simulink model "LKA_RL_staliro"  (R2021a)
settings: Solver=FixedStepAuto  StartTime=0.0  StopTime=T  FixedStep=Ts  RelTol=1e-3
undefined symbols (not defined in the file): Cf, Cr, DiscIntNeverNeededParam, e1_initial, e2_initial, Iz, lf, lr, m, max_late_dev, md, terminate_error, Ts, u_max, u_min, Vx
libraries: rllib x1, simulink x1
settings Model: Creator=The MathWorks, Inc.  LastModifiedBy=ldy
settings SolverCC: AlgebraicLoopSolver=TrustRegion
settings DataIOCC: ReturnWorkspaceOutputs=off
settings DebuggingCC: SFMachineParentedDataDiag=warning  ArithmeticOperatorsInVariantConditions=warning
settings SFSimCC: SimUseLocalCustomCode=off  CustomCodeUndefinedFunction=UseInterfaceOnly
settings RTWCC: RTWUseLocalCustomCode=off
settings CodeAppCC: StateflowObjectComments=on
settings SimscapeCC: SimscapeNormalizeSystem=off

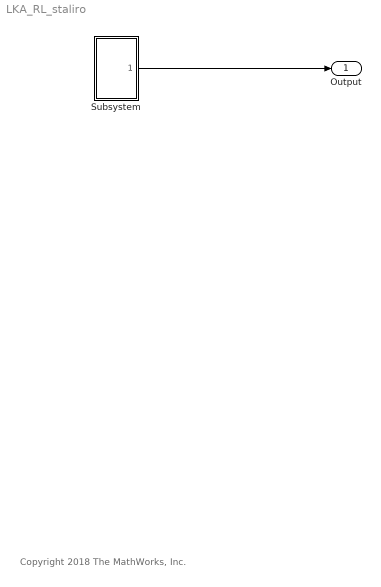
== system LKA_RL_staliro ==
  note: Copyright 2018 The MathWorks, Inc.
  Subsystem : Subsystem
  Output : Outport
  wires:
  Subsystem/1(Outport) -> Output/1

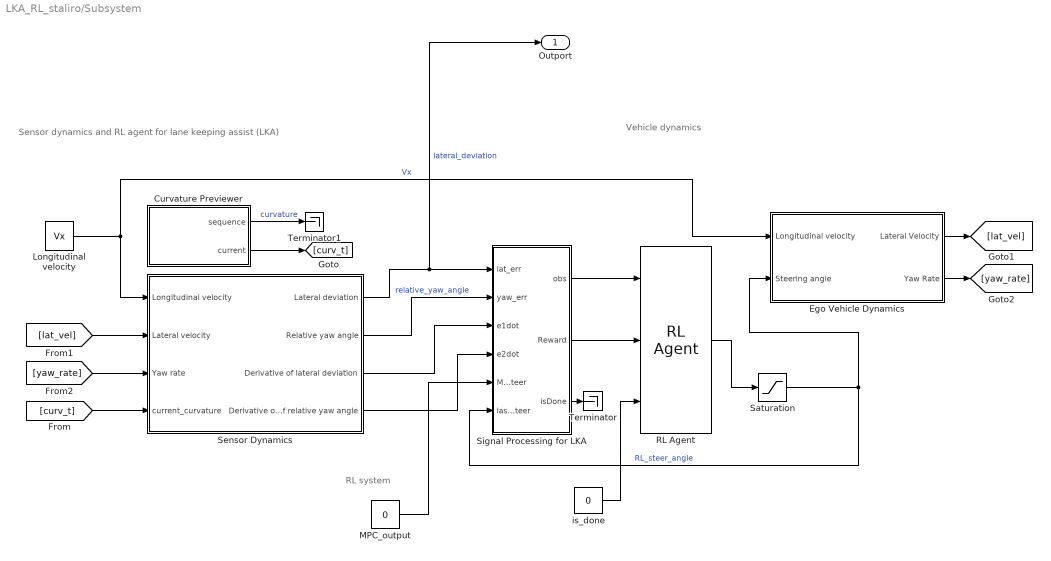
== system LKA_RL_staliro/Subsystem ==
  note: RL system
  note: Vehicle dynamics
  note: Sensor dynamics and RL agent for lane keeping assist (LKA)
  Curvature Previewer : Subsystem  mask{signal=md, ts=Ts, steps=10}
      mask prompts: signal "Signal name"; ts "Sampling time"; steps "Number of previewing steps"
      mask init:
      | ts = evalin('base',get_param(gcbh,'ts'));
      | signal = evalin('base',get_param(gcbh,'signal'));
      | steps = evalin('base',get_param(gcbh,'steps'));
      | data = mpc_previewer_maskinit(signal,ts);
      mask Display:
      | fprintf('Future\nsample\nextractor');
      | port_label('output', 1, 'seq')
      | port_label('output', 2, '@t')
  Ego Vehicle Dynamics : Subsystem
  Longitudinal velocity : Constant  Value=Vx  SampleTime=Ts
  MPC_output : Constant  Value=0
  RL Agent : rllib/RL Agent  Agent=agent  ExternalActionAsInput=off  ProvideCumRwd=off  TreatAsDirectFeedthrough=on
  Saturation : Saturate  UpperLimit=u_max  LowerLimit=u_min
  Sensor Dynamics : Subsystem
  "Signal Processing for LKA " : Subsystem
  Terminator : Terminator
  Terminator1 : Terminator
  is_done : Constant  Value=0
  Outport : Outport
  wires:
  Curvature Previewer/2(current) -> [curv_t]
  [curv_t] -> Sensor Dynamics/4(current_curvature)
  Curvature Previewer/1(sequence) -> Terminator1/1  "curvature"
  [yaw_rate] -> Sensor Dynamics/3(Yaw rate)
  Ego Vehicle Dynamics/1(Lateral Velocity) -> [lat_vel]
  MPC_output/1 -> "Signal Processing for LKA "/5(MPC_steer)
  is_done/1 -> RL Agent/3
  Sensor Dynamics/3(Derivative of lateral deviation) -> "Signal Processing for LKA "/3("e1dot ")
  "Signal Processing for LKA "/2(Reward) -> RL Agent/2
  Sensor Dynamics/1(Lateral deviation) -> Outport/1, "Signal Processing for LKA "/1(lat_err)  "lateral_deviation"
  RL Agent/1 -> Saturation/1
  "Signal Processing for LKA "/1(obs) -> RL Agent/1
  Sensor Dynamics/4(Derivative of relative yaw angle) -> "Signal Processing for LKA "/4(e2dot)
  [lat_vel] -> Sensor Dynamics/2(Lateral velocity)
  Saturation/1 -> "Signal Processing for LKA "/6(last_RL_steer), Ego Vehicle Dynamics/2(Steering angle)  "RL_steer_angle"
  Sensor Dynamics/2(Relative yaw angle) -> "Signal Processing for LKA "/2(yaw_err)  "relative_yaw_angle"
  Ego Vehicle Dynamics/2(Yaw Rate) -> [yaw_rate]
  Longitudinal velocity/1 -> Ego Vehicle Dynamics/1(Longitudinal velocity), Sensor Dynamics/1(Longitudinal velocity)  "Vx"
  "Signal Processing for LKA "/3(isDone) -> Terminator/1

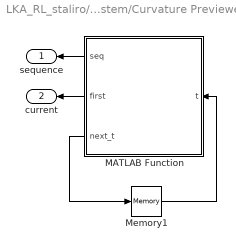
== system LKA_RL_staliro/Subsystem/Curvature Previewer ==
  MATLAB Function : MATLAB Function  TreatAsAtomicUnit=on
  Memory1 : Memory  InheritSampleTime=on  LinearizeAsDelay=on
  sequence : Outport  VectorParamsAs1DForOutWhenUnconnected=off
  current : Outport  Port=2  VectorParamsAs1DForOutWhenUnconnected=off
  wires:
  MATLAB Function/1(seq) -> sequence/1
  MATLAB Function/2(first) -> current/1
  Memory1/1 -> MATLAB Function/1(t)
  MATLAB Function/3(next_t) -> Memory1/1

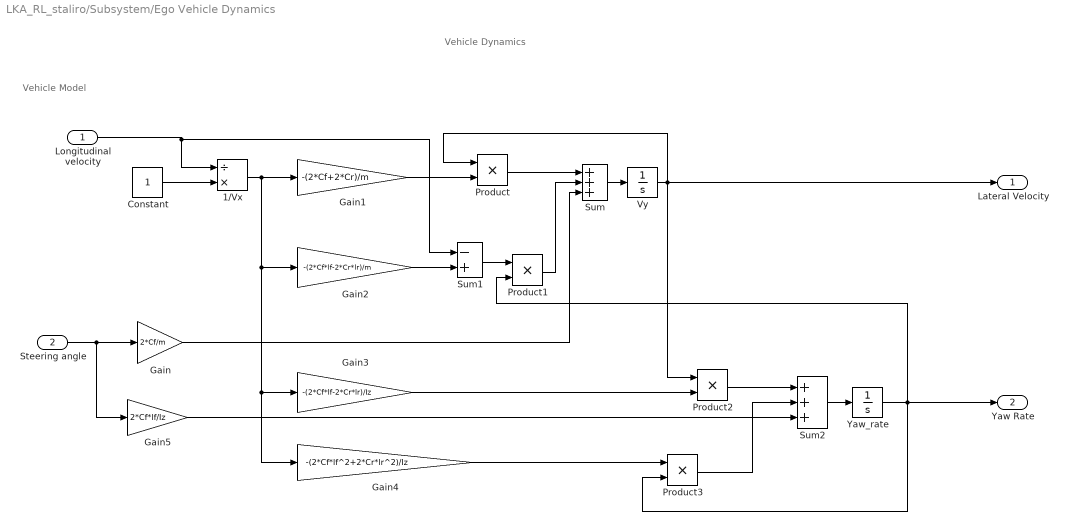
== system LKA_RL_staliro/Subsystem/Ego Vehicle Dynamics ==
  note: Vehicle Model
  note: Vehicle Dynamics
  Longitudinal velocity : Inport
  Steering angle : Inport  Port=2
  1/Vx : Product  Inputs=/*
  Constant : Constant
  Gain : Gain  Gain=2*Cf/m
  Gain1 : Gain  Gain=-(2*Cf+2*Cr)/m
  Gain2 : Gain  Gain=-(2*Cf*lf-2*Cr*lr)/m
  Gain3 : Gain  Gain=-(2*Cf*lf-2*Cr*lr)/Iz
  Gain4 : Gain  Gain=-(2*Cf*lf^2+2*Cr*lr^2)/Iz
  Gain5 : Gain  Gain=2*Cf*lf/Iz
  Product{,1..3} (4 alike) : Product
  Sum : Sum  Inputs=+++
  Sum1 : Sum  Inputs=-+
  Sum2 : Sum  Inputs=+++
  Vy : Integrator
  "Yaw_rate " : Integrator
  Lateral Velocity : Outport  VectorParamsAs1DForOutWhenUnconnected=off
  Yaw Rate : Outport  Port=2  VectorParamsAs1DForOutWhenUnconnected=off
  wires:
  Sum2/1 -> "Yaw_rate "/1
  Gain2/1 -> Sum1/2
  Gain4/1 -> Product3/1
  Constant/1 -> 1/Vx/2
  Gain3/1 -> Product2/2
  1/Vx/1 -> Gain4/1, Gain3/1, Gain2/1, Gain1/1
  Product2/1 -> Sum2/1
  Product3/1 -> Sum2/2
  Gain5/1 -> Sum2/3
  Sum1/1 -> Product1/1
  "Yaw_rate "/1 -> Product3/2, Yaw Rate/1, Product1/2
  Gain/1 -> Sum/3
  Steering angle/1 -> Gain/1, Gain5/1
  Gain1/1 -> Product/2
  Product/1 -> Sum/1
  Vy/1 -> Product/1, Lateral Velocity/1, Product2/1
  Sum/1 -> Vy/1
  Longitudinal velocity/1 -> Sum1/1, 1/Vx/1
  Product1/1 -> Sum/2

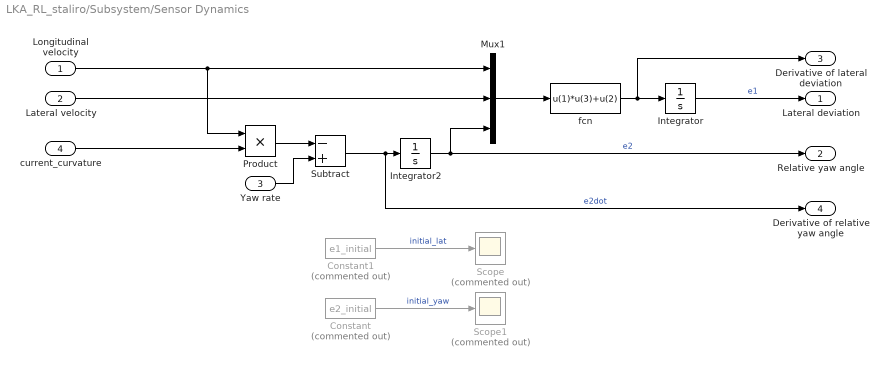
== system LKA_RL_staliro/Subsystem/Sensor Dynamics ==
  Longitudinal velocity : Inport
  Lateral velocity : Inport  Port=2
  Yaw rate : Inport  Port=3
  current_curvature : Inport  Port=4
  Constant : Constant  Commented=on  Value=e2_initial
  Constant1 : Constant  Commented=on  Value=e1_initial
  Integrator : Integrator  InitialCondition=e1_initial
  Integrator2 : Integrator  InitialCondition=e2_initial
  Mux1 : Mux  Inputs=[1 1 1]
  Product : Product
  Scope : Scope  Commented=on
  Scope1 : Scope  Commented=on
  Subtract : Sum  Inputs=-+
  fcn : Fcn  Expr=u(1)*u(3)+u(2)
  Lateral deviation : Outport  VectorParamsAs1DForOutWhenUnconnected=off
  Relative yaw angle : Outport  Port=2  VectorParamsAs1DForOutWhenUnconnected=off
  Derivative of lateral deviation : Outport  Port=3  VectorParamsAs1DForOutWhenUnconnected=off
  Derivative of relative yaw angle : Outport  Port=4  VectorParamsAs1DForOutWhenUnconnected=off
  wires:
  Integrator2/1 -> Relative yaw angle/1, Mux1/3  "e2"
  Mux1/1 -> fcn/1
  fcn/1 -> Derivative of lateral deviation/1, Integrator/1
  Lateral velocity/1 -> Mux1/2
  Integrator/1 -> Lateral deviation/1  "e1"
  Product/1 -> Subtract/1
  Yaw rate/1 -> Subtract/2
  Subtract/1 -> Derivative of relative yaw angle/1, Integrator2/1  "e2dot"
  Longitudinal velocity/1 -> Mux1/1, Product/1
  current_curvature/1 -> Product/2
  Constant1/1 -> Scope/1  "initial_lat"
  Constant/1 -> Scope1/1  "initial_yaw"

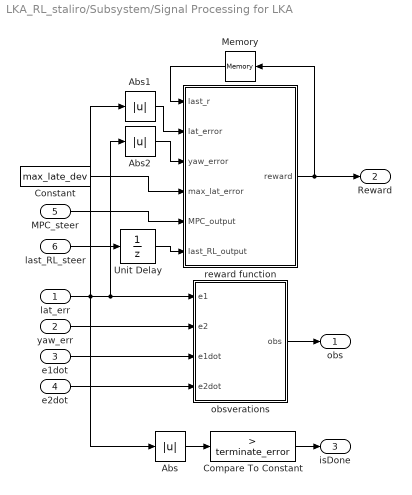
== system LKA_RL_staliro/Subsystem/Signal Processing for LKA  ==
  lat_err : Inport
  yaw_err : Inport  Port=2
  "e1dot " : Inport  Port=3
  e2dot : Inport  Port=4
  MPC_steer : Inport  Port=5
  last_RL_steer : Inport  Port=6
  Abs : Abs
  Abs1 : Abs
  Abs2 : Abs
  Compare To Constant : simulink/Logic and Bit Operations/Compare To Constant  relop=>  const=terminate_error  OutDataTypeStr=boolean
  Constant : Constant  Value=max_late_dev
  Memory : Memory
  Unit Delay : UnitDelay  SampleTime=-1  HasFrameUpgradeWarning=on
  obsverations : Subsystem
  reward function : MATLAB Function  TreatAsAtomicUnit=on
  obs : Outport  VectorParamsAs1DForOutWhenUnconnected=off
  Reward : Outport  Port=2  VectorParamsAs1DForOutWhenUnconnected=off
  isDone : Outport  Port=3  VectorParamsAs1DForOutWhenUnconnected=off
  wires:
  Abs/1 -> Compare To Constant/1
  Compare To Constant/1 -> isDone/1
  obsverations/1(obs) -> obs/1
  "e1dot "/1 -> obsverations/3(e1dot)
  e2dot/1 -> obsverations/4(e2dot)
  yaw_err/1 -> obsverations/2(e2)
  lat_err/1 -> Abs1/1, Abs/1, Abs2/1, obsverations/1(e1)
  reward function/1(reward) -> Memory/1, Reward/1
  Constant/1 -> reward function/4(max_lat_error)
  Abs1/1 -> reward function/2(lat_error)
  Abs2/1 -> reward function/3(yaw_error)
  MPC_steer/1 -> reward function/5(MPC_output)
  last_RL_steer/1 -> Unit Delay/1
  Unit Delay/1 -> reward function/6(last_RL_output)
  Memory/1 -> reward function/1(last_r)

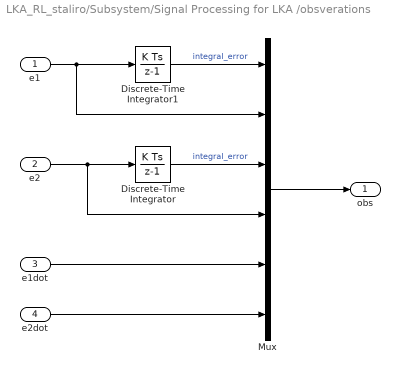
== system LKA_RL_staliro/Subsystem/Signal Processing for LKA /obsverations ==
  e1 : Inport
  e2 : Inport  Port=2
  e1dot : Inport  Port=3
  e2dot : Inport  Port=4
  Discrete-Time Integrator : DiscreteIntegrator  SampleTime=-1  ICPrevOutput=DiscIntNeverNeededParam  ICPrevScaledInput=DiscIntNeverNeededParam
  Discrete-Time Integrator1 : DiscreteIntegrator  SampleTime=-1  ICPrevOutput=DiscIntNeverNeededParam  ICPrevScaledInput=DiscIntNeverNeededParam
  Mux : Mux  Inputs=6
  obs : Outport  VectorParamsAs1DForOutWhenUnconnected=off
  wires:
  e1/1 -> Mux/2, Discrete-Time Integrator1/1
  Mux/1 -> obs/1
  Discrete-Time Integrator1/1 -> Mux/1  "integral_error"
  e2/1 -> Mux/4, Discrete-Time Integrator/1
  Discrete-Time Integrator/1 -> Mux/3  "integral_error"
  e1dot/1 -> Mux/5
  e2dot/1 -> Mux/6

== matlab function LKA_RL_staliro/Subsystem/Signal Processing for LKA /reward function ==
  data: last_r input; lat_error input; reward output; yaw_error input; max_lat_error input; MPC_output input; last_RL_output input
function reward = fcn(last_r, lat_error, yaw_error, max_lat_error, MPC_output, last_RL_output)

% pos_reward = 0.7*exp(-(lat_error*3)^2) + 0.3*exp(-(yaw_error*2)^2);
% 
% MPC_reward = 0.1*exp(-((last_RL_output - MPC_output)*15)^2);
% 
% last_steer_reward = -0.05*tanh(abs(last_RL_output)*6);
% 
% if lat_error >= max_lat_error
%     neg_reward = -tanh((lat_error- max_lat_error)*15);
% else
%     neg_reward = -0.3*tanh(lat_error*5);
% end
% 
% reward = pos_reward + neg_reward + MPC_reward;

pos_reward = exp(-(lat_error*3)^2) + exp(-(yaw_error*2)^2);

MPC_reward = 0.1*exp(-((last_RL_output - MPC_output)*15)^2);

last_steer_reward = -0.05*tanh(abs(last_RL_output)*6);

if lat_error >= max_lat_error
    neg_reward = -2*tanh((lat_error- max_lat_error)*15);
else
    neg_reward = -0.5*tanh(lat_error*5);
end

reward = pos_reward + neg_reward;

% MSR algorithm
r_p = reward + 1e-8;
last_r_p = last_r + 1e-8;

rho = (r_p - last_r_p)/min(abs(r_p), abs(last_r_p));
lambda = sign(r_p - last_r_p);
x = rho + lambda;
eta = 5;
f_x = atan(x*pi/2*1/eta);

if x > eta
    reward = r_p + (f_x - lambda)*abs(r_p);
end

== matlab function LKA_RL_staliro/Subsystem/Curvature Previewer/MATLAB Function ==
  settings: updateMethod=DISCRETE  sampleTime=ts
  data: data parameter; seq output; steps parameter; t input; first output; next_t output
function [seq,first,next_t] = fcn(data,steps,t)
%#codegen
[seq,first,next_t] = mpcblock_preview('md',data,steps,t);
